simulink model "dsp_project_nonstationary"  (R2024b)
settings: Solver=VariableStepAuto  StartTime=0.0  StopTime=10.0  RelTol=1e-3
values from neighbouring files (symbols this model uses):
  b = (sqrt(1+4*t_frames^2)-1)/(2*t_frames^2)    [dsp_project_nonstaion.m]
  Lf = max(1, round(freq_mask_smooth_hz / (fs/nfft)))    [dsp_project_matalb.m]    (also in dsp_project_nonstaion.m)
  Lt = max(1, round(time_mask_smooth_ms / (hop/fs*1e3)))    [dsp_project_matalb.m]    (also in dsp_project_nonstaion.m)
  prop = 0.9    [dsp_project_nonstaion.m]
  sigmoid_slope = 10    [dsp_project_nonstaion.m]
  thresh_n_mult_nonstationary = 0.9    [dsp_project_nonstaion.m]
undefined symbols (not defined in the file or in its folder): dspblkCoreblockFVToolHelper, gcbh
libraries: dspvision x3, dspxfrm3 x2, dspsigops x1
settings Model: Creator=settlab  LastModifiedBy=settlab

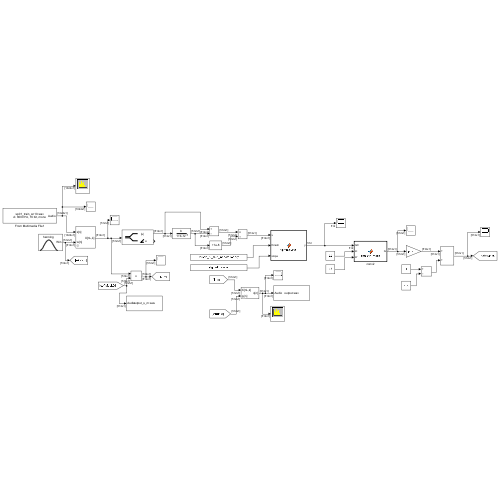
[thumbnail: Simulink's stored preview of the top-level diagram]
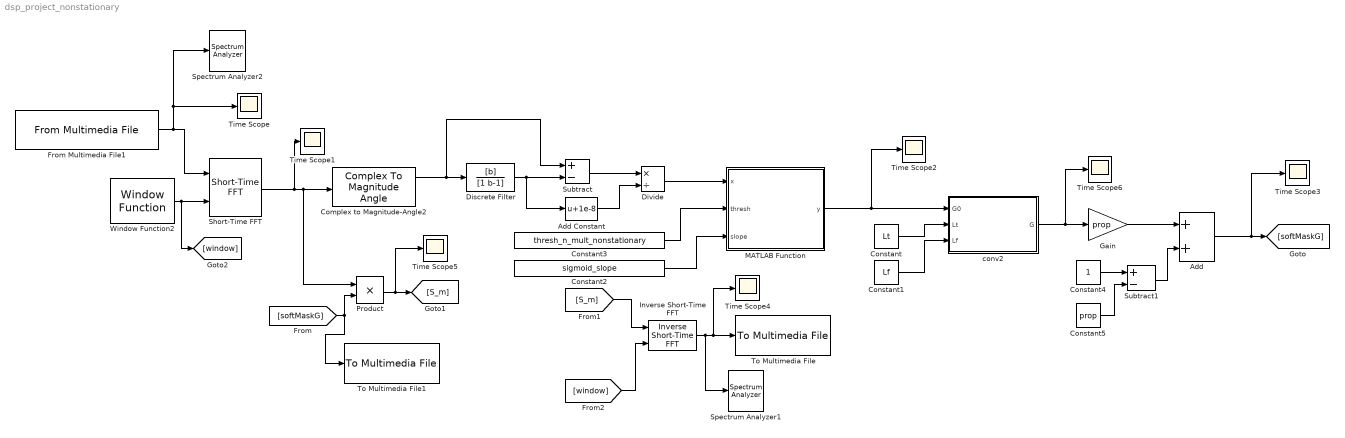
== system dsp_project_nonstationary ==
  Add : Sum
  Add Constant : Bias  Bias=1e-8  SaturateOnIntegerOverflow=off
  Complex to Magnitude-Angle2 : ComplexToMagnitudeAngle
  Constant : Constant  Value=Lt
  Constant1 : Constant  Value=Lf
  Constant2 : Constant  Value=sigmoid_slope
  Constant3 : Constant  Value=thresh_n_mult_nonstationary
  Constant4 : Constant
  Constant5 : Constant  Value=prop
  Discrete Filter : DiscreteFilter  LoadFcn=dspblkCoreblockFVToolHelper(gcbh,'load');  Numerator=[b]  Denominator=[1 b-1]
      settings: CopyFcn=dspblkCoreblockFVToolHelper(gcbh,'copy');  DeleteFcn=dspblkCoreblockFVToolHelper(gcbh,'close');  ModelCloseFcn=dspblkCoreblockFVToolHelper(gcbh,'close');  PreSaveFcn=dspblkCoreblockFVToolHelper(gcbh,'presave');  PostSaveFcn=dspblkCoreblockFVToolHelper(gcbh,'postsave');  CloseFcn=dspblkCoreblockFVToolHelper(gcbh,'close');
  Divide : Product  Inputs=*/
  From Multimedia File1 : dspvision/From Multimedia File  inputFilename=C:\Users\settlab\Downloads\sp01_train_sn10.wav  readRange=[1 Inf]  loop=on  numPlays=inf  outputStreams=오디오 전용  videoDataType=single  audioDataType=double  inheritSampleTime=on  userDefinedSampleTime=fs  noAudioOutput=off  isIntensityVideo=off  fourcc=RGB  colorVideoFormat=One multidimensional signal  outputEOF=off  dataOrg=Column-major  audioFrameSize=1024  computeAudioFrameSize=off  outSamplingMode=Sample based
      settings: LibrarySourceBlock=dspsrcs4/From Multimedia File
  Gain : Gain  Gain=prop
  Inverse Short-Time FFT : dspxfrm3/Inverse  Short-Time FFT  W=512  OvLap=378  OutFrameSize=512  InConjSymm=on  DoAssert=off  Tol=1e-4  OutputFrames=off
  MATLAB Function : MATLAB Function  TreatAsAtomicUnit=on
  Product : Product
  Short-Time FFT : dspxfrm3/Short-Time FFT  W=512  OvLap=378  M=512
  Spectrum Analyzer1 : SpectrumAnalyzer  WindowPosition=[1093.000000,523.000000,800.000000,500.000000,]  ScopeFrameLocation=window  ViewType=Spectrum and spectrogram  Method=Welch  PlotAsTwoSidedSpectrum=off  AveragingMethod=Exponential  YLimits=[-93.52641013,-13.53435914]  ColorLimits=[-93.52641013,-13.53435914]
  Spectrum Analyzer2 : SpectrumAnalyzer  WindowPosition=[277.000000,522.000000,800.000000,500.000000,]  ScopeFrameLocation=window  ViewType=Spectrum and spectrogram  Method=Welch  PlotAsTwoSidedSpectrum=off  AveragingMethod=Exponential  YLimits=[-108.43759021,1.67136395]  ColorLimits=[-108.43759021,1.67136395]
  Subtract : Sum  Inputs=+-
  Subtract1 : Sum  Inputs=+-
  Time Scope{,1..6} (7 alike) : Scope
  To Multimedia File : dspvision/To Multimedia File  outputFilename=C:\Users\settlab\Documents\MATLAB\EIS_SSG\output.wav  streamSelection=Audio only  videoCompressor=None (uncompressed)  audioCompressor=None (uncompressed)  imagePorts=One multidimensional signal  fileType=WAV  audioDatatype=16-bit integer  fourcc=RGB  audioBitRate=128  audioQuality=75  videoQuality=75  mj2000CompFactor=10
      settings: LibrarySourceBlock=dspsnks4/To Multimedia File
  To Multimedia File1 : dspvision/To Multimedia File  outputFilename=C:\Users\settlab\Documents\MATLAB\EIS_SSG\output_s_m.wav  streamSelection=Audio only  videoCompressor=None (uncompressed)  audioCompressor=None (uncompressed)  imagePorts=One multidimensional signal  fileType=WAV  audioDatatype=16-bit integer  fourcc=RGB  audioBitRate=128  audioQuality=75  videoQuality=75  mj2000CompFactor=10
      settings: LibrarySourceBlock=dspsnks4/To Multimedia File
  Window Function2 : dspsigops/Window Function  winmode=Generate window  wintype=Hanning  sampmode=Discrete  samptime=-1  N=512  Rs=50  beta=10  winsamp=Symmetric  UserWindow=hamming  OptParams=off  UserParams={'symmetric'}  dataType=double  isSigned=on  wordLen=16  udDataType=sfix(16)  fracBitsMode=Best precision  numFracBits=15  roundingMode=Floor  overflowMode=off  numSidelobes=4  sidelobeLevel=-30
  conv2 : MATLAB Function  TreatAsAtomicUnit=on
  wires:
  Inverse Short-Time FFT/1 -> Spectrum Analyzer1/1, Time Scope4/1, To Multimedia File/1
  From Multimedia File1/1 -> Spectrum Analyzer2/1, Time Scope/1, Short-Time FFT/1
  [softMaskG] -> Product/2, To Multimedia File1/1
  Product/1 -> Time Scope5/1, [S_m]
  [window] -> Inverse Short-Time FFT/2
  Short-Time FFT/1 -> Time Scope1/1, Product/1, Complex to Magnitude-Angle2/1
  [S_m] -> Inverse Short-Time FFT/1
  Window Function2/1 -> [window], Short-Time FFT/2
  Discrete Filter/1 -> Add Constant/1, Subtract/2
  Complex to Magnitude-Angle2/1 -> Subtract/1, Discrete Filter/1
  Subtract/1 -> Divide/1
  Divide/1 -> MATLAB Function/1(x)
  Constant2/1 -> MATLAB Function/3(slope)
  Constant3/1 -> MATLAB Function/2(thresh)
  MATLAB Function/1(y) -> Time Scope2/1, conv2/1(G0)
  Constant/1 -> conv2/2(Lt)
  Constant1/1 -> conv2/3(Lf)
  conv2/1(G) -> Time Scope6/1, Gain/1
  Gain/1 -> Add/1
  Constant4/1 -> Subtract1/1
  Subtract1/1 -> Add/2
  Constant5/1 -> Subtract1/2
  Add/1 -> Time Scope3/1, [softMaskG]
  Add Constant/1 -> Divide/2

== matlab function dsp_project_nonstationary/MATLAB Function ==
  data: x input; y output; thresh input; slope input
function y = sigmoidMask(x, thresh, slope)
%#codegen
y = 1 ./ (1 + exp(-slope*(x - thresh)));
end

== matlab function dsp_project_nonstationary/conv2 ==
  data: G0 input; G output; Lt input; Lf input
function G = smooth_mask(G0, Lt, Lf)
%#codegen
% G0 : [M×N] double matrix
% Lt, Lf : positive integer kernel lengths

    %=== 1) 입력 유효성 검사 ===
    assert(isnumeric(G0) && ndims(G0)==2, ...
        'smooth_mask: G0 must be a 2D numeric matrix');
    assert(isscalar(Lt) && Lt>=1 && Lt==round(Lt), ...
        'smooth_mask: Lt must be a positive integer scalar');
    assert(isscalar(Lf) && Lf>=1 && Lf==round(Lf), ...
        'smooth_mask: Lf must be a positive integer scalar');

    %=== 2) Lt=Lf=1 이면 패스스루 ===
    if Lt==1 && Lf==1
        G = G0;
        return;
    end

    %=== 3) 삼각 커널 생성 ===
    % triang 이 codegen에서 지원되지 않을 수도 있으니, 직접 만들어 봅니다.
    kt = 1:Lt;
    kt = min(kt, Lt-(kt-1));    % [1 2 ... ceil(Lt/2) ... 2 1]
    kf = 1:Lf;
    kf = min(kf, Lf-(kf-1));    % [1 2 ... ceil(Lf/2) ... 2 1]

    %=== 4) 정규화 계수 계산 ===
    sum_kt = sum(kt);
    sum_kf = sum(kf);
    normFactor = sum_kt * sum_kf;  % Σ(kt)*Σ(kf)

    %=== 5) 분리형 2D 컨볼루션 ===
    % vert conv: each column마다 kt
    Gtmp = conv2(G0, kt(:), 'same');
    % horz conv: 각 행마다 kf
    Gtmp = conv2(Gtmp, kf(:).', 'same');

    %=== 6) 정규화 ===
    G = Gtmp ./ normFactor;
end
